simulink model "model"  (R2018b)
settings: Solver=ode4  StartTime=0.0  StopTime=10.0  FixedStep=1e-2  RelTol=1e-3
values from neighbouring files (symbols this model uses):
  A = 1    [Basics.m]
  f = 1/T    (= 10)    [Basics.m]
  K = 1/(R*C)    (= 6.66666666667)    [Basics.m]
  s1 = 3    [Basics.m]
  s2 = 0    [Basics.m]
  ts = 5    [Basics.m]
  WPC = 3    [Basics.m]
settings Model: Creator=bion  LastModifiedBy=bion

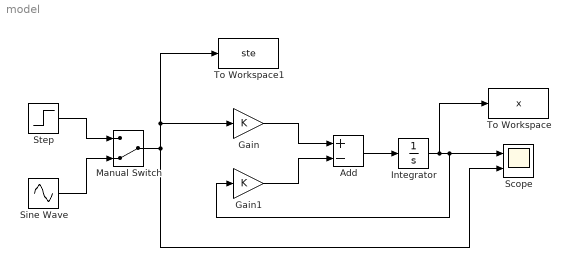
== system model ==
  Add : Sum  Inputs=+-
  Gain : Gain  Gain=K
  Gain1 : Gain  Gain=K
  Integrator : Integrator  InitialCondition=WPC
  Manual Switch : ManualSwitch  CurrentSetting=0
  Scope : Scope  NumInputPorts=2
  Sine Wave : Sin  Amplitude=A  Frequency=f  SampleTime=0
  Step : Step  Time=ts  Before=s1  After=s2  SampleTime=0
  To Workspace : ToWorkspace  VariableName=x  SampleTime=-1
  To Workspace1 : ToWorkspace  VariableName=ste  SampleTime=-1
  wires:
  Sine Wave/1 -> Manual Switch/2
  Step/1 -> Manual Switch/1
  Gain1/1 -> Add/2
  Gain/1 -> Add/1
  Add/1 -> Integrator/1
  Integrator/1 -> Gain1/1, Scope/1, To Workspace/1
  Manual Switch/1 -> Scope/2, To Workspace1/1, Gain/1
